simulink model "filter_bank_1"  (Simulink 5.1)
settings: Solver=ode45  StartTime=0.0  StopTime=1  RelTol=1e-3
values from neighbouring files (symbols this model uses):
  nf = 256    [band4.m]    (also in block_lms_.m = 16)
undefined symbols (not defined in the file or in its folder): cos_m
libraries: dspbuff3 x1, dspsigattribs x1
settings Model: Creator=svenhoffmann  LastModifiedBy=svenhoffmann  ExtModeAutoUpdateStatusClock=off  BooleanDataType=on  ProdHWDeviceType=Microprocessor

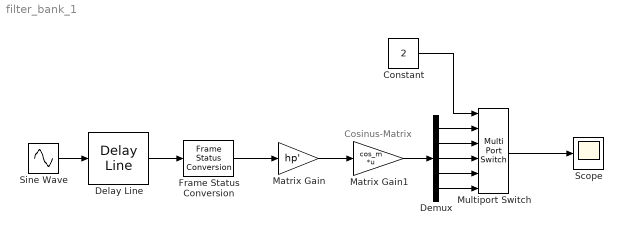
== system filter_bank_1 ==
  note: Cosinus-Matrix
  Constant : Constant  Value=2
  Delay Line : dspbuff3/Delay Line  siz=nf+1  ic=0  directfeed=off
  Demux : Demux  Outputs=5
  Frame Status Conversion : dspsigattribs/Frame Status Conversion  growRefPort=off  outframe=Sample-based
  Matrix Gain : Gain  Gain=hp'  SaturateOnIntegerOverflow=on
  Matrix Gain1 : Gain  Gain=cos_m  Multiplication=Matrix(K*u)  SaturateOnIntegerOverflow=on
  Multiport Switch : MultiPortSwitch  Inputs=5  SaturateOnIntegerOverflow=on
  Scope : Scope
  Sine Wave : Sin  Frequency=2*pi*100  SampleTime=1/1000
  wires:
  Sine Wave/1 -> Delay Line/1
  Delay Line/1 -> Frame Status Conversion/1
  Matrix Gain/1 -> Matrix Gain1/1
  Matrix Gain1/1 -> Demux/1
  Demux/1 -> Multiport Switch/2
  Demux/2 -> Multiport Switch/3
  Demux/3 -> Multiport Switch/4
  Demux/4 -> Multiport Switch/5
  Demux/5 -> Multiport Switch/6
  Constant/1 -> Multiport Switch/1
  Multiport Switch/1 -> Scope/1
  Frame Status Conversion/1 -> Matrix Gain/1
